simulink model "libraryALL"  (Simulink 7.9)
settings: Solver=ode45  StartTime=0.0  StopTime=10.0  RelTol=1e-3
libraries: dspmtrx3 x2, dspsolvers x1
settings Model: Creator=jorhabib  LastModifiedBy=jorhabib

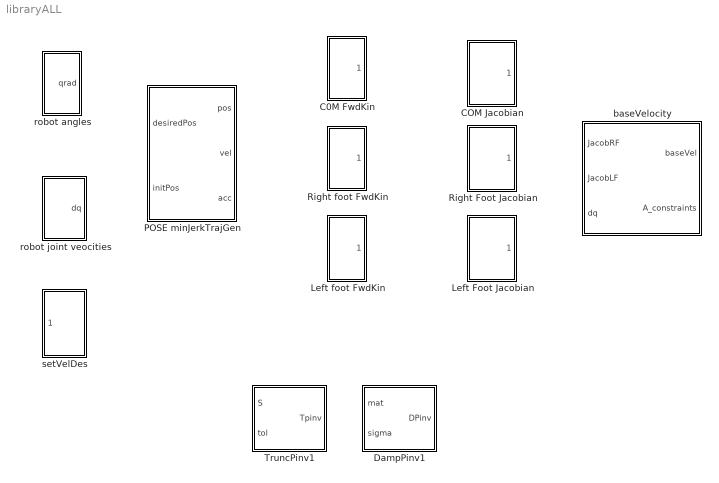
== system libraryALL ==
  C0M FwdKin : Subsystem
  COM Jacobian : Subsystem
  DampPinv1 : Subsystem  mask{tol=1e-4}
      mask prompts: tol "Tolerance"
  Left Foot Jacobian : Subsystem
  Left foot FwdKin : Subsystem
  POSE minJerkTrajGen : Subsystem
  Right Foot Jacobian : Subsystem
  Right foot FwdKin : Subsystem
  TruncPinv1 : Subsystem  mask{tol=1e-4}
      mask prompts: tol "Tolerance"
  baseVelocity : Subsystem
  robot angles : Subsystem
  robot joint veocities : Subsystem
  setVelDes : Subsystem

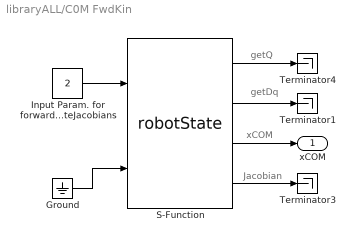
== system libraryALL/C0M FwdKin ==
  note: getDq
  note: xCOM
  note: getQ
  note: Jacobian
  Ground : Ground
  "Input Param. for forwardKinematics and  computeJacobians " : Constant  Value=2  OutDataTypeStr=int8
  S-Function : S-Function  FunctionName=robotState  Parameters=val,robotname,localname  EnableBusSupport=off  mask{val=2, robotname='icubSim', localname='robotState'}
      mask prompts: val "Value"; robotname "Robot Name (icub - icubSim)"; localname "Module Name"
  Terminator1 : Terminator
  Terminator3 : Terminator
  Terminator4 : Terminator
  xCOM : Outport
  wires:
  Ground/1 -> S-Function/2
  S-Function/2 -> Terminator1/1
  S-Function/1 -> Terminator4/1
  S-Function/3 -> xCOM/1
  "Input Param. for forwardKinematics and  computeJacobians "/1 -> S-Function/1
  S-Function/4 -> Terminator3/1

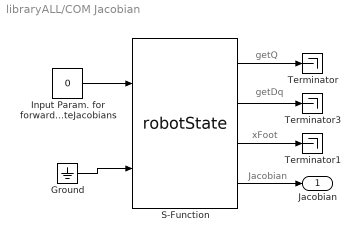
== system libraryALL/COM Jacobian ==
  note: Jacobian
  note: getQ
  note: xFoot
  note: getDq
  Ground : Ground
  "Input Param. for forwardKinematics and  computeJacobians " : Constant  Value=0  OutDataTypeStr=int8
  S-Function : S-Function  FunctionName=robotState  Parameters=val,robotname,localname  EnableBusSupport=off  mask{val=3, robotname='icubSim', localname='robotState'}
      mask prompts: val "Value"; robotname "Robot Name (icub - icubSim)"; localname "Module Name"
  Terminator : Terminator
  Terminator1 : Terminator
  Terminator3 : Terminator
  Jacobian : Outport
  wires:
  S-Function/4 -> Jacobian/1
  "Input Param. for forwardKinematics and  computeJacobians "/1 -> S-Function/1
  S-Function/3 -> Terminator1/1
  S-Function/1 -> Terminator/1
  S-Function/2 -> Terminator3/1
  Ground/1 -> S-Function/2

== system libraryALL/DampPinv1 ==
  mat : Inport
  sigma : Inport  Port=2
  Damped Pseudo Inverse : MATLAB Function  TreatAsAtomicUnit=on
  DPinv : Outport
  wires:
  mat/1 -> Damped Pseudo Inverse/1(mat)
  Damped Pseudo Inverse/1(DPinv) -> DPinv/1
  sigma/1 -> Damped Pseudo Inverse/2(sigma)

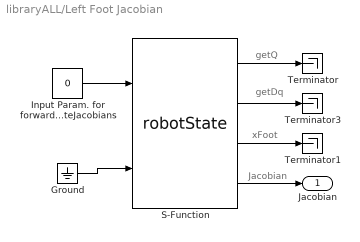
== system libraryALL/Left Foot Jacobian ==
  note: Jacobian
  note: getQ
  note: xFoot
  note: getDq
  Ground : Ground
  "Input Param. for forwardKinematics and  computeJacobians " : Constant  Value=0  OutDataTypeStr=int8
  S-Function : S-Function  FunctionName=robotState  Parameters=val,robotname,localname  EnableBusSupport=off  mask{val=3, robotname='icubSim', localname='robotState'}
      mask prompts: val "Value"; robotname "Robot Name (icub - icubSim)"; localname "Module Name"
  Terminator : Terminator
  Terminator1 : Terminator
  Terminator3 : Terminator
  Jacobian : Outport
  wires:
  S-Function/4 -> Jacobian/1
  "Input Param. for forwardKinematics and  computeJacobians "/1 -> S-Function/1
  S-Function/3 -> Terminator1/1
  S-Function/1 -> Terminator/1
  S-Function/2 -> Terminator3/1
  Ground/1 -> S-Function/2

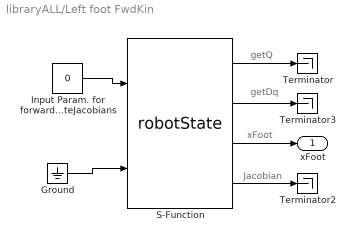
== system libraryALL/Left foot FwdKin ==
  note: Jacobian
  note: getQ
  note: xFoot
  note: getDq
  Ground : Ground
  "Input Param. for forwardKinematics and  computeJacobians " : Constant  Value=0  OutDataTypeStr=int8
  S-Function : S-Function  FunctionName=robotState  Parameters=val,robotname,localname  EnableBusSupport=off  mask{val=2, robotname='icubSim', localname='robotState'}
      mask prompts: val "Value"; robotname "Robot Name (icub - icubSim)"; localname "Module Name"
  Terminator : Terminator
  Terminator2 : Terminator
  Terminator3 : Terminator
  xFoot : Outport
  wires:
  Ground/1 -> S-Function/2
  S-Function/4 -> Terminator2/1
  "Input Param. for forwardKinematics and  computeJacobians "/1 -> S-Function/1
  S-Function/3 -> xFoot/1
  S-Function/1 -> Terminator/1
  S-Function/2 -> Terminator3/1

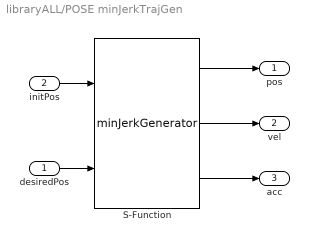
== system libraryALL/POSE minJerkTrajGen ==
  desiredPos : Inport
  initPos : Inport  Port=2
  S-Function : S-Function  FunctionName=minJerkGenerator  Parameters=dim, rate, tt  EnableBusSupport=off  mask{dim=25, rate=10, tt=4}
      mask prompts: dim "Trajectory dimension (int)"; rate "Simulation rate (int) [ms]"; tt "Trajectory time [s]"
  pos : Outport
  vel : Outport  Port=2
  acc : Outport  Port=3
  wires:
  S-Function/2 -> vel/1
  S-Function/1 -> pos/1
  S-Function/3 -> acc/1
  initPos/1 -> S-Function/1
  desiredPos/1 -> S-Function/2

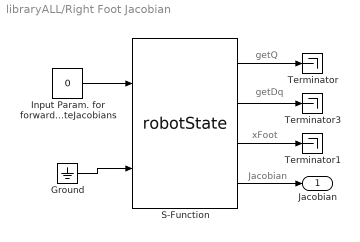
== system libraryALL/Right Foot Jacobian ==
  note: getDq
  note: xFoot
  note: getQ
  note: Jacobian
  Ground : Ground
  "Input Param. for forwardKinematics and  computeJacobians " : Constant  Value=0  OutDataTypeStr=int8
  S-Function : S-Function  FunctionName=robotState  Parameters=val,robotname,localname  EnableBusSupport=off  mask{val=3, robotname='icubSim', localname='robotState'}
      mask prompts: val "Value"; robotname "Robot Name (icub - icubSim)"; localname "Module Name"
  Terminator : Terminator
  Terminator1 : Terminator
  Terminator3 : Terminator
  Jacobian : Outport
  wires:
  Ground/1 -> S-Function/2
  S-Function/2 -> Terminator3/1
  S-Function/1 -> Terminator/1
  S-Function/3 -> Terminator1/1
  "Input Param. for forwardKinematics and  computeJacobians "/1 -> S-Function/1
  S-Function/4 -> Jacobian/1

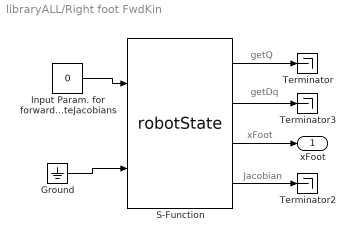
== system libraryALL/Right foot FwdKin ==
  note: getDq
  note: xFoot
  note: getQ
  note: Jacobian
  Ground : Ground
  "Input Param. for forwardKinematics and  computeJacobians " : Constant  Value=0  OutDataTypeStr=int8
  S-Function : S-Function  FunctionName=robotState  Parameters=val,robotname,localname  EnableBusSupport=off  mask{val=2, robotname='icubSim', localname='robotState'}
      mask prompts: val "Value"; robotname "Robot Name (icub - icubSim)"; localname "Module Name"
  Terminator : Terminator
  Terminator2 : Terminator
  Terminator3 : Terminator
  xFoot : Outport
  wires:
  S-Function/2 -> Terminator3/1
  S-Function/1 -> Terminator/1
  S-Function/3 -> xFoot/1
  "Input Param. for forwardKinematics and  computeJacobians "/1 -> S-Function/1
  S-Function/4 -> Terminator2/1
  Ground/1 -> S-Function/2

== system libraryALL/TruncPinv1 ==
  S : Inport
  tol : Inport  Port=2
  Truncated PseudoInverse : MATLAB Function  TreatAsAtomicUnit=on
  Tpinv : Outport
  wires:
  tol/1 -> Truncated PseudoInverse/2(tol)
  Truncated PseudoInverse/1(TPinv) -> Tpinv/1
  S/1 -> Truncated PseudoInverse/1(mat)

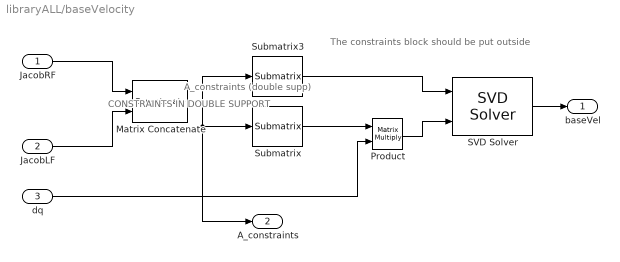
== system libraryALL/baseVelocity ==
  note: The constraints block should be put outside
  note: CONSTRAINTS IN DOUBLE SUPPORT
  note: A_constraints
      | (double supp)
  JacobRF : Inport
  JacobLF : Inport  Port=2
  dq : Inport  Port=3
  Matrix Concatenate : Concatenate  Mode=Multidimensional array
  Product : Product  Multiplication=Matrix(*)  RndMeth=Zero
  SVD Solver : dspsolvers/SVD Solver  wanterr=off
  Submatrix : dspmtrx3/Submatrix  RowSpan=Range of rows  RowStartMode=First  RowStartIndex=1  RowEndMode=Last  RowEndIndex=1  ColSpan=Range of columns  ColStartMode=Index  ColStartIndex=7  ColEndMode=Last  ColEndIndex=1
  Submatrix3 : dspmtrx3/Submatrix  RowSpan=Range of rows  RowStartMode=First  RowStartIndex=1  RowEndMode=Last  RowEndIndex=1  ColSpan=Range of columns  ColStartMode=First  ColStartIndex=7  ColEndMode=Index  ColEndIndex=6
  baseVel : Outport
  A_constraints : Outport  Port=2
  wires:
  Matrix Concatenate/1 -> A_constraints/1, Submatrix/1, Submatrix3/1
  Submatrix3/1 -> SVD Solver/1
  JacobRF/1 -> Matrix Concatenate/1
  SVD Solver/1 -> baseVel/1
  JacobLF/1 -> Matrix Concatenate/2
  Submatrix/1 -> Product/1
  Product/1 -> SVD Solver/2
  dq/1 -> Product/2

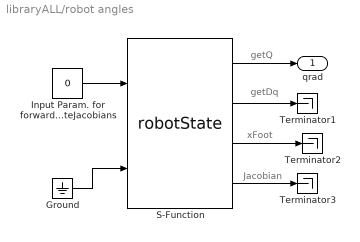
== system libraryALL/robot angles ==
  note: Jacobian
  note: getQ
  note: xFoot
  note: getDq
  Ground : Ground
  "Input Param. for forwardKinematics and  computeJacobians " : Constant  Value=0  OutDataTypeStr=int8
  S-Function : S-Function  FunctionName=robotState  Parameters=val,robotname,localname  EnableBusSupport=off  mask{val=0, robotname='icubSim', localname='robotState'}
      mask prompts: val "Value"; robotname "Robot Name (icub - icubSim)"; localname "Module Name"
  Terminator1 : Terminator
  Terminator2 : Terminator
  Terminator3 : Terminator
  qrad : Outport
  wires:
  S-Function/4 -> Terminator3/1
  "Input Param. for forwardKinematics and  computeJacobians "/1 -> S-Function/1
  S-Function/3 -> Terminator2/1
  S-Function/1 -> qrad/1
  S-Function/2 -> Terminator1/1
  Ground/1 -> S-Function/2

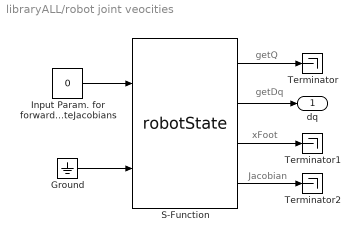
== system libraryALL/robot joint veocities ==
  note: Jacobian
  note: getQ
  note: xFoot
  note: getDq
  Ground : Ground
  "Input Param. for forwardKinematics and  computeJacobians " : Constant  Value=0  OutDataTypeStr=int8
  S-Function : S-Function  FunctionName=robotState  Parameters=val,robotname,localname  EnableBusSupport=off  mask{val=1, robotname='icubSim', localname='robotState'}
      mask prompts: val "Value"; robotname "Robot Name (icub - icubSim)"; localname "Module Name"
  Terminator : Terminator
  Terminator1 : Terminator
  Terminator2 : Terminator
  dq : Outport
  wires:
  S-Function/4 -> Terminator2/1
  "Input Param. for forwardKinematics and  computeJacobians "/1 -> S-Function/1
  S-Function/3 -> Terminator1/1
  S-Function/1 -> Terminator/1
  S-Function/2 -> dq/1
  Ground/1 -> S-Function/2

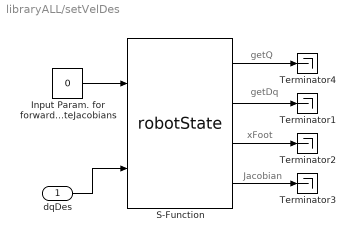
== system libraryALL/setVelDes ==
  note: getDq
  note: xFoot
  note: getQ
  note: Jacobian
  dqDes : Inport
  "Input Param. for forwardKinematics and  computeJacobians " : Constant  Value=0  OutDataTypeStr=int8
  S-Function : S-Function  FunctionName=robotState  Parameters=val,robotname,localname  EnableBusSupport=off  mask{val=4, robotname='icubSim', localname='robotState'}
      mask prompts: val "Value"; robotname "Robot Name (icub - icubSim)"; localname "Module Name"
  Terminator{1..4} (4 alike) : Terminator
  wires:
  dqDes/1 -> S-Function/2
  S-Function/2 -> Terminator1/1
  S-Function/1 -> Terminator4/1
  S-Function/3 -> Terminator2/1
  "Input Param. for forwardKinematics and  computeJacobians "/1 -> S-Function/1
  S-Function/4 -> Terminator3/1

== matlab function DampPinv1/Damped Pseudo Inverse ==
  data: mat input double; DPinv output double; sigma input double
function DPinv  = fcn(mat,sigma)
% Economody size svd of mat
[U,S,V] = svd(mat,'econ');
% Damped version of S with sigma
S(S>sigma)=S(S>sigma)./((S(S>sigma)).^2+sigma^2);
% Damped pseudoinverse
DPinv = V*pinv(S)*U';

== matlab function TruncPinv1/Truncated PseudoInverse ==
  data: mat input double; TPinv output double; tol input double
function TPinv  = fcn(mat,tol)
%#codegen
[U,S,V] = svd(mat,'econ');
% Setting to zero value
% Setting to 1/S(i,i) singular values greater than tol
 S(S>tol)=1./S(S>tol);
 TPinv = V*pinv(S)*U';
